simulink model "untitled1"  (R2020b)
settings: Solver=ode45  StartTime=0.0  StopTime=ts  MaxStep=0.1  RelTol=1e-3
values from neighbouring files (symbols this model uses):
  ax = ks*cos(Theta_T)-3*x_T    [Praca_magisterska.m]
  ay = ks*sin(Theta_T)-3*y_T    [Praca_magisterska.m]
  e = [(beta_T - beta_0);(Theta_T - Theta_0 - (g*beta_0*T));     (y_T - y_0 - g*Theta_0*T - (0.5*g^2*beta_0*T^2))]    [Praca_magisterska.m]
  l = 0.5    [Praca_magisterska.m]
  m = 0.5    [Praca_magisterska.m]
  r = 0.2    [Praca_magisterska.m]
  tp = tp*2    (= 24000)    [Praca_magisterska.m]
  X = [X X1]    [Praca_magisterska.m]    (also in myfile.m = t13.*t26.*x_0+t.*t13.*x_T-(t.*t14.*t26.*t28)./2.0; spoly.m = -t31.*t57-t37.*t55-t50.*x_0+t7.*t22.*x_T)
  Y = [Y Y1]    [Praca_magisterska.m]    (also in myfile.m = y_0-t9.*((t13.*t48)./2.0+t14.*t50.*4.0+t15.*t49.*1.0e+1)+t10; spoly.m = -t31.*t58-t37.*t56-t50.*y_0+t7.*t22.*y_T)
settings Model: Creator=gumia  LastModifiedBy=gumia
settings SolverCC: MaxConsecutiveMinStep=2  AlgebraicLoopSolver=LineSearch

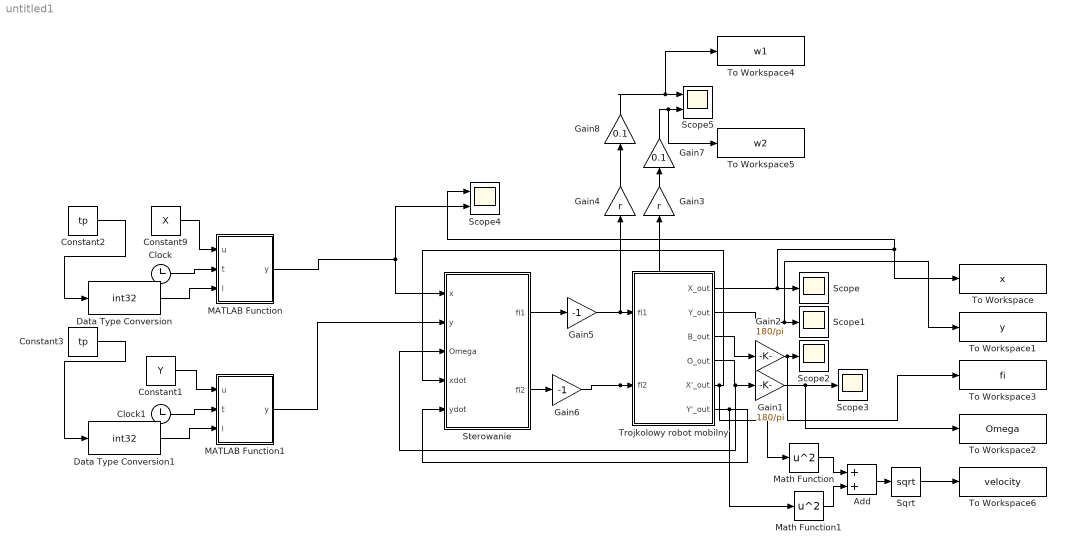
== system untitled1 ==
  Add : Sum
  Clock : Clock
  Clock1 : Clock
  Constant1 : Constant  Value=Y
  Constant2 : Constant  Value=tp
  Constant3 : Constant  Value=tp
  Constant9 : Constant  Value=X
  Data Type Conversion : DataTypeConversion  OutDataTypeStr=int32
  Data Type Conversion1 : DataTypeConversion  OutDataTypeStr=int32
  Gain1 : Gain  Gain=180/pi
  Gain2 : Gain  Gain=180/pi
  Gain3 : Gain  Gain=r
  Gain4 : Gain  Gain=r
  Gain5 : Gain  Gain=-1
  Gain6 : Gain  Gain=-1
  Gain7 : Gain  Gain=0.1
  Gain8 : Gain  Gain=0.1
  MATLAB Function : MATLAB Function  TreatAsAtomicUnit=on
  MATLAB Function1 : MATLAB Function  TreatAsAtomicUnit=on
  Math Function : Math  Operator=square  SaturateOnIntegerOverflow=on
  Math Function1 : Math  Operator=square  SaturateOnIntegerOverflow=on
  Scope{,1..3} (4 alike) : Scope
  Scope4 : Scope  NumInputPorts=2
  Scope5 : Scope  NumInputPorts=2
  Sqrt : Sqrt  SaturateOnIntegerOverflow=on
  Sterowanie : Subsystem
  To Workspace : ToWorkspace  VariableName=x  SampleTime=-1
      settings: Save2DSignal=2-D array (concatenate along first dimension)
  To Workspace1 : ToWorkspace  VariableName=y  SampleTime=-1
      settings: Save2DSignal=2-D array (concatenate along first dimension)
  To Workspace2 : ToWorkspace  VariableName=Omega  SampleTime=-1
      settings: Save2DSignal=2-D array (concatenate along first dimension)
  To Workspace3 : ToWorkspace  VariableName=fi  SampleTime=-1
      settings: Save2DSignal=2-D array (concatenate along first dimension)
  To Workspace4 : ToWorkspace  VariableName=w1  SampleTime=-1
      settings: Save2DSignal=2-D array (concatenate along first dimension)
  To Workspace5 : ToWorkspace  VariableName=w2  SampleTime=-1
      settings: Save2DSignal=2-D array (concatenate along first dimension)
  To Workspace6 : ToWorkspace  VariableName=velocity  SampleTime=-1
      settings: Save2DSignal=2-D array (concatenate along first dimension)
  Trojkolowy robot mobilny : Subsystem  mask{r=r, l=l, m=m, e=e}
      mask prompts: r "Promien kola napedowego"; l "Szerokosc modelu"; m "Odleglosc osi od kola sterowego"; e "Odleglosc osi od punktu sledzenia traj"
  wires:
  Sterowanie/1("fi1 ") -> Gain5/1
  Sterowanie/2(fi2) -> Gain6/1
  Trojkolowy robot mobilny/1(X_out) -> To Workspace/1, Scope4/1, Scope/1
  Trojkolowy robot mobilny/3(B_out) -> Gain2/1
  Gain2/1 -> To Workspace3/1, Scope2/1
  Trojkolowy robot mobilny/4(O_out) -> Gain1/1, Sterowanie/3(Omega)
  Trojkolowy robot mobilny/6(Y'_out) -> Math Function1/1, Sterowanie/5("ydot ")
  Trojkolowy robot mobilny/5(X'_out) -> Math Function/1, Sterowanie/4(xdot)
  Trojkolowy robot mobilny/2(Y_out) -> To Workspace1/1, Scope1/1
  Constant2/1 -> Data Type Conversion/1
  Data Type Conversion/1 -> MATLAB Function/3(l)
  Clock/1 -> MATLAB Function/2(t)
  Constant3/1 -> Data Type Conversion1/1
  Data Type Conversion1/1 -> MATLAB Function1/3(l)
  Clock1/1 -> MATLAB Function1/2(t)
  MATLAB Function1/1(y) -> Sterowanie/2("y ")
  MATLAB Function/1(y) -> Sterowanie/1(x), Scope4/2
  Gain4/1 -> Gain8/1
  Gain3/1 -> Gain7/1
  Gain1/1 -> Scope3/1, To Workspace2/1
  Gain5/1 -> Gain4/1, Trojkolowy robot mobilny/1(fi1)
  Gain6/1 -> Gain3/1, Trojkolowy robot mobilny/2("fi2 ")
  Constant1/1 -> MATLAB Function1/1(u)
  Constant9/1 -> MATLAB Function/1(u)
  Math Function/1 -> Add/1
  Math Function1/1 -> Add/2
  Add/1 -> Sqrt/1
  Sqrt/1 -> To Workspace6/1
  Gain8/1 -> To Workspace4/1, Scope5/1
  Gain7/1 -> To Workspace5/1, Scope5/2

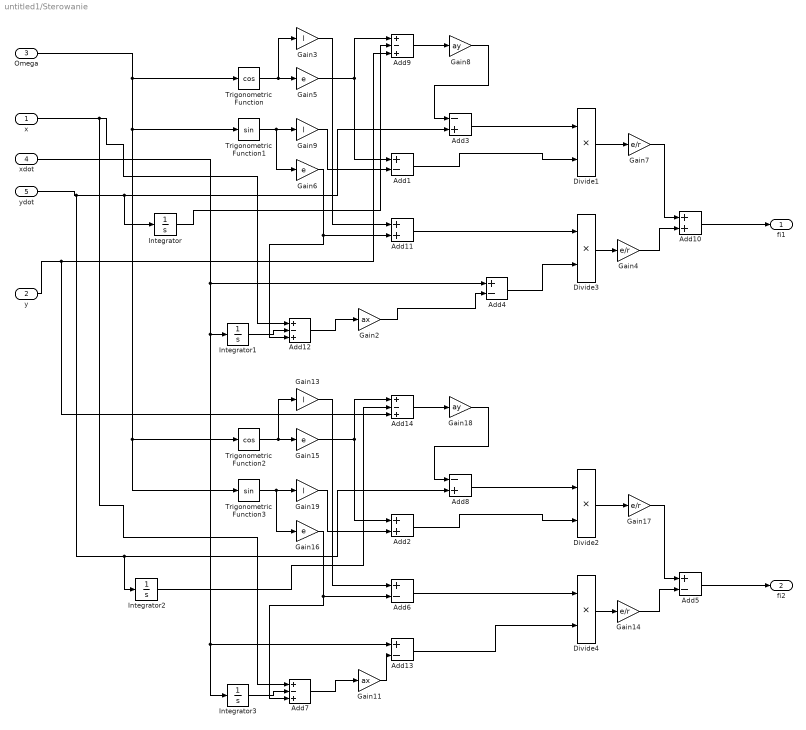
== system untitled1/Sterowanie ==
  x : Inport
  "y " : Inport  Port=2
  Omega : Inport  Port=3
  xdot : Inport  Port=4
  "ydot " : Inport  Port=5
  Add{1,4..6,13} (5 alike) : Sum  Inputs=+-
  Add10 : Sum
  Add11 : Sum
  Add{7,9,12,14} (4 alike) : Sum  Inputs=+-+
  Add2 : Sum
  Add3 : Sum  Inputs=-+
  Add8 : Sum  Inputs=-+
  Divide{1..4} (4 alike) : Product  Inputs=**
  Gain11 : Gain  Gain=ax
  Gain{3,9,13,19} (4 alike) : Gain  Gain=l
  Gain{4,7,14,17} (4 alike) : Gain  Gain=e/r
  Gain{5..6,15..16} (4 alike) : Gain  Gain=e
  Gain18 : Gain  Gain=ay
  Gain2 : Gain  Gain=ax
  Gain8 : Gain  Gain=ay
  Integrator{,1..3} (4 alike) : Integrator
  Trigonometric Function : Trigonometry  Operator=cos
  Trigonometric Function1 : Trigonometry
  Trigonometric Function2 : Trigonometry  Operator=cos
  Trigonometric Function3 : Trigonometry
  "fi1 " : Outport
  fi2 : Outport  Port=2
  wires:
  Trigonometric Function/1 -> Gain3/1, Gain5/1
  Gain5/1 -> Add1/1, Add9/1
  Integrator/1 -> Add9/2
  Add9/1 -> Gain8/1
  Gain8/1 -> Add3/1
  Add3/1 -> Divide1/1
  Trigonometric Function1/1 -> Gain6/1, Gain9/1
  Gain9/1 -> Add1/2
  Gain6/1 -> Add12/3, Add11/2
  Gain3/1 -> Add11/1
  Add1/1 -> Divide1/2
  Divide1/1 -> Gain7/1
  Gain7/1 -> Add10/1
  Add11/1 -> Divide3/1
  Integrator1/1 -> Add12/2
  Add12/1 -> Gain2/1
  Add4/1 -> Divide3/2
  Divide3/1 -> Gain4/1
  Gain4/1 -> Add10/2
  Add10/1 -> "fi1 "/1
  Omega/1 -> Trigonometric Function/1, Trigonometric Function1/1, Trigonometric Function3/1, Trigonometric Function2/1
  Add2/1 -> Divide2/2
  Gain19/1 -> Add2/2
  Gain18/1 -> Add8/1
  Trigonometric Function2/1 -> Gain13/1, Gain15/1
  Gain15/1 -> Add2/1, Add14/1
  Gain11/1 -> Add13/2
  Divide2/1 -> Gain17/1
  Add6/1 -> Divide4/1
  xdot/1 -> Add13/1, Integrator3/1, Integrator1/1, Add4/1
  Add8/1 -> Divide2/1
  "ydot "/1 -> Add8/2, Integrator2/1, Add3/2, Integrator/1
  Gain17/1 -> Add5/1
  Gain16/1 -> Add7/3, Add6/2
  x/1 -> Add7/1, Add12/1
  Add14/1 -> Gain18/1
  "y "/1 -> Add14/3, Add9/3
  Gain13/1 -> Add6/1
  Trigonometric Function3/1 -> Gain16/1, Gain19/1
  Divide4/1 -> Gain14/1
  Add7/1 -> Gain11/1
  Integrator3/1 -> Add7/2
  Add5/1 -> fi2/1
  Gain14/1 -> Add5/2
  Integrator2/1 -> Add14/2
  Add13/1 -> Divide4/2
  Gain2/1 -> Add4/2

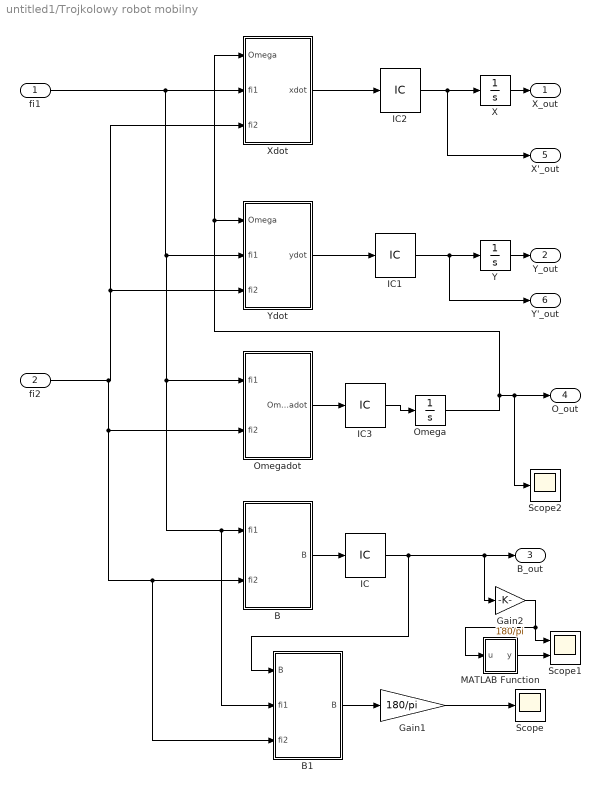
== system untitled1/Trojkolowy robot mobilny ==
  fi1 : Inport
  "fi2 " : Inport  Port=2
  B : Subsystem
  B1 : Subsystem
  Gain1 : Gain  Gain=180/pi
  Gain2 : Gain  Gain=180/pi
  IC{,1..3} (4 alike) : InitialCondition  Value=0
  MATLAB Function : MATLAB Function  TreatAsAtomicUnit=on
  Omega : Integrator
  Omegadot : Subsystem
  Scope : Scope
  Scope1 : Scope  NumInputPorts=2
  Scope2 : Scope
  X : Integrator
  Xdot : Subsystem
  Y : Integrator
  Ydot : Subsystem
  X_out : Outport
  Y_out : Outport  Port=2
  B_out : Outport  Port=3
  O_out : Outport  Port=4
  X'_out : Outport  Port=5
  Y'_out : Outport  Port=6
  wires:
  B/1("B ") -> IC/1
  Xdot/1("xdot ") -> IC2/1
  IC1/1 -> Y'_out/1, Y/1
  Ydot/1("ydot ") -> IC1/1
  fi1/1 -> B1/2(fi1), B/1(fi1), Omegadot/1(fi1), Ydot/2(fi1), Xdot/2(fi1)
  Y/1 -> Y_out/1
  IC2/1 -> X'_out/1, X/1
  X/1 -> X_out/1
  "fi2 "/1 -> B1/3("fi2 "), B/2("fi2 "), Omegadot/2("fi2 "), Ydot/3("fi2 "), Xdot/3("fi2 ")
  B1/1("B ") -> Gain1/1
  Gain1/1 -> Scope/1
  Gain2/1 -> MATLAB Function/1(u), Scope1/1
  IC/1 -> B1/1(B), B_out/1, Gain2/1
  MATLAB Function/1(y) -> Scope1/2
  Omegadot/1("Omegadot ") -> IC3/1
  Omega/1 -> Scope2/1, O_out/1, Xdot/1(Omega), Ydot/1(Omega)
  IC3/1 -> Omega/1

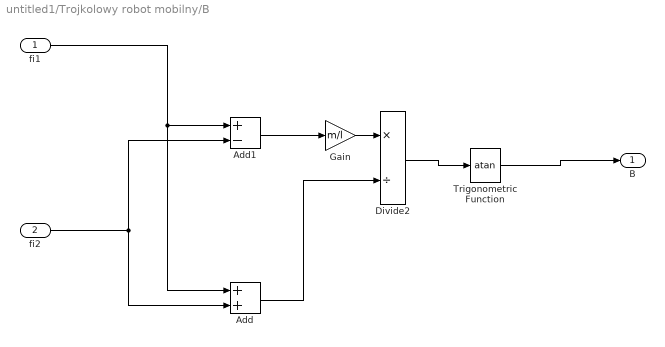
== system untitled1/Trojkolowy robot mobilny/B ==
  fi1 : Inport
  "fi2 " : Inport  Port=2
  Add : Sum
  Add1 : Sum  Inputs=+-
  Divide2 : Product  Inputs=*/
  Gain : Gain  Gain=m/l
  Trigonometric Function : Trigonometry  Operator=atan
  "B " : Outport
  wires:
  "fi2 "/1 -> Add1/2, Add/2
  Add1/1 -> Gain/1
  Divide2/1 -> Trigonometric Function/1
  Gain/1 -> Divide2/1
  Add/1 -> Divide2/2
  fi1/1 -> Add1/1, Add/1
  Trigonometric Function/1 -> "B "/1

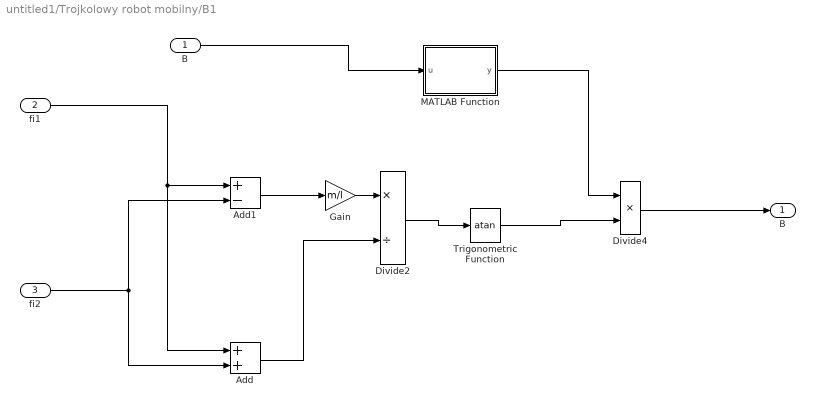
== system untitled1/Trojkolowy robot mobilny/B1 ==
  B : Inport
  fi1 : Inport  Port=2
  "fi2 " : Inport  Port=3
  Add : Sum
  Add1 : Sum  Inputs=+-
  Divide2 : Product  Inputs=*/
  Divide4 : Product  Inputs=**
  Gain : Gain  Gain=m/l
  MATLAB Function : MATLAB Function  TreatAsAtomicUnit=on
  Trigonometric Function : Trigonometry  Operator=atan
  "B " : Outport
  wires:
  B/1 -> MATLAB Function/1(u)
  MATLAB Function/1(y) -> Divide4/1
  Divide4/1 -> "B "/1
  Add/1 -> Divide2/2
  fi1/1 -> Add1/1, Add/1
  Trigonometric Function/1 -> Divide4/2
  Add1/1 -> Gain/1
  Divide2/1 -> Trigonometric Function/1
  Gain/1 -> Divide2/1
  "fi2 "/1 -> Add1/2, Add/2

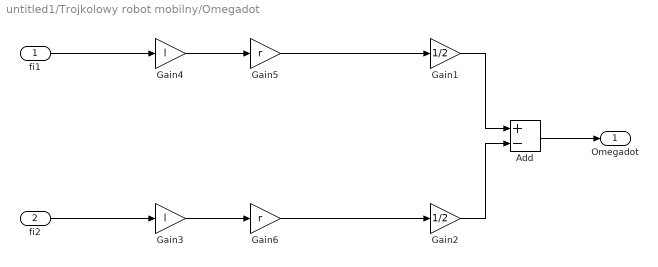
== system untitled1/Trojkolowy robot mobilny/Omegadot ==
  fi1 : Inport
  "fi2 " : Inport  Port=2
  Add : Sum  Inputs=+-
  Gain1 : Gain  Gain=1/2
  Gain2 : Gain  Gain=1/2
  Gain3 : Gain  Gain=l
  Gain4 : Gain  Gain=l
  Gain5 : Gain  Gain=r
  Gain6 : Gain  Gain=r
  "Omegadot " : Outport
  wires:
  Add/1 -> "Omegadot "/1
  fi1/1 -> Gain4/1
  "fi2 "/1 -> Gain3/1
  Gain3/1 -> Gain6/1
  Gain2/1 -> Add/2
  Gain1/1 -> Add/1
  Gain4/1 -> Gain5/1
  Gain5/1 -> Gain1/1
  Gain6/1 -> Gain2/1

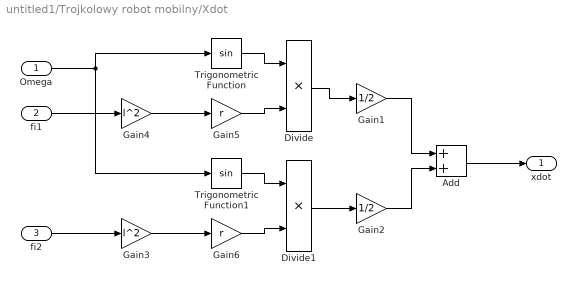
== system untitled1/Trojkolowy robot mobilny/Xdot ==
  Omega : Inport
  fi1 : Inport  Port=2
  "fi2 " : Inport  Port=3
  Add : Sum
  Divide : Product  Inputs=**
  Divide1 : Product  Inputs=**
  Gain1 : Gain  Gain=1/2
  Gain2 : Gain  Gain=1/2
  Gain3 : Gain  Gain=l^2
  Gain4 : Gain  Gain=l^2
  Gain5 : Gain  Gain=r
  Gain6 : Gain  Gain=r
  Trigonometric Function : Trigonometry
  Trigonometric Function1 : Trigonometry
  "xdot " : Outport
  wires:
  Omega/1 -> Trigonometric Function1/1, Trigonometric Function/1
  Trigonometric Function1/1 -> Divide1/1
  Trigonometric Function/1 -> Divide/1
  Add/1 -> "xdot "/1
  fi1/1 -> Gain4/1
  Divide1/1 -> Gain2/1
  Gain2/1 -> Add/2
  Divide/1 -> Gain1/1
  Gain1/1 -> Add/1
  Gain4/1 -> Gain5/1
  Gain5/1 -> Divide/2
  Gain3/1 -> Gain6/1
  Gain6/1 -> Divide1/2
  "fi2 "/1 -> Gain3/1

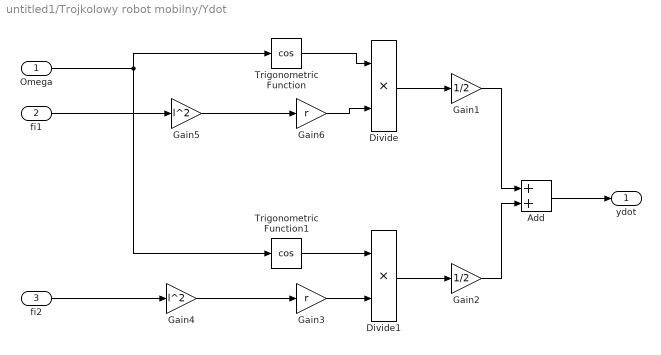
== system untitled1/Trojkolowy robot mobilny/Ydot ==
  Omega : Inport
  fi1 : Inport  Port=2
  "fi2 " : Inport  Port=3
  Add : Sum
  Divide : Product  Inputs=**
  Divide1 : Product  Inputs=**
  Gain1 : Gain  Gain=1/2
  Gain2 : Gain  Gain=1/2
  Gain3 : Gain  Gain=r
  Gain4 : Gain  Gain=l^2
  Gain5 : Gain  Gain=l^2
  Gain6 : Gain  Gain=r
  Trigonometric Function : Trigonometry  Operator=cos
  Trigonometric Function1 : Trigonometry  Operator=cos
  "ydot " : Outport
  wires:
  Trigonometric Function1/1 -> Divide1/1
  Trigonometric Function/1 -> Divide/1
  Omega/1 -> Trigonometric Function/1, Trigonometric Function1/1
  Add/1 -> "ydot "/1
  Divide1/1 -> Gain2/1
  Gain2/1 -> Add/2
  Divide/1 -> Gain1/1
  Gain1/1 -> Add/1
  fi1/1 -> Gain5/1
  Gain5/1 -> Gain6/1
  Gain6/1 -> Divide/2
  "fi2 "/1 -> Gain4/1
  Gain4/1 -> Gain3/1
  Gain3/1 -> Divide1/2

== matlab function untitled1/MATLAB Function ==
  data: u input; y output; t input; l input
function y = fcn(u,t,l)


if l >= int32(t*10+1)

    x = u(int32(t*10+1));
    
else
    
   x =u(end);
end
y = x;

== matlab function untitled1/Trojkolowy robot mobilny/B1/MATLAB Function ==
  data: u input; y output
function y = fcn(u)
y = sign(u);
y = u;

== matlab function untitled1/Trojkolowy robot mobilny/MATLAB Function ==
  data: u input; y output
function y = fcn(u)
windowSize = 5; 
b = (1/windowSize)*ones(1,windowSize);
a = 0.5;
k = filter(b,a,u);
y = k;

== matlab function untitled1/MATLAB Function1 ==
  data: u input; y output; t input; l input
function y = fcn(u,t,l)
 
if l >= int32(t*10+1)

    x = u(int32(t*10+1));
    
else
    
   x =u(end);
end
y = x;
